simulink model "modele"  (R2016b)
settings: Solver=VariableStepAuto  StartTime=0.0  StopTime=2  RelTol=1e-3
values from neighbouring files (symbols this model uses):
  f = 0    [data_modele.m]
  Jeq = J0*Km^2    (= 3.4375e-05)    [data_modele.m]
  Ke = (1/182)*(30/pi)    (= 0.0524686625578)    [data_modele.m]
  Km = 25*1e-3    (= 0.025)    [data_modele.m]
  Kp = 200    [data_modele.m]
  Kt = 52.5*1e-3    (= 0.0525)    [data_modele.m]
  L = 0.62*1e-3    (= 0.00062)    [data_modele.m]
  R = 2.07    [data_modele.m]
settings Model: Creator=emiliendurif  LastModifiedBy=emiliendurif

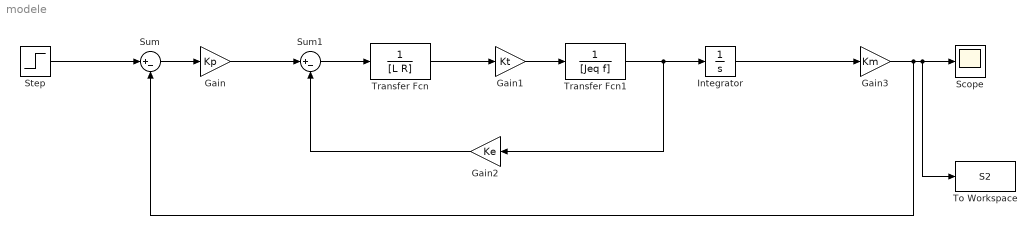
== system modele ==
  Gain : Gain  Gain=Kp
  Gain1 : Gain  Gain=Kt
  Gain2 : Gain  Gain=Ke
  Gain3 : Gain  Gain=Km
  Integrator : Integrator
  Scope : Scope
  Step : Step  Time=0  After=20  SampleTime=0  ZeroCross=off
  Sum : Sum  Inputs=|+-
  Sum1 : Sum  Inputs=|+-
  To Workspace : ToWorkspace  VariableName=S2  SaveFormat=Timeseries  SampleTime=-1
  Transfer Fcn : TransferFcn  Denominator=[L R]
  Transfer Fcn1 : TransferFcn  Denominator=[Jeq f]
  wires:
  Sum/1 -> Gain/1
  Gain/1 -> Sum1/1
  Gain2/1 -> Sum1/2
  Sum1/1 -> Transfer Fcn/1
  Transfer Fcn/1 -> Gain1/1
  Gain1/1 -> Transfer Fcn1/1
  Transfer Fcn1/1 -> Gain2/1, Integrator/1
  Integrator/1 -> Gain3/1
  Gain3/1 -> Sum/2, To Workspace/1, Scope/1
  Step/1 -> Sum/1
